simulink model "cruise_model_expanded"  (R2017a)
settings: Solver=VariableStepAuto  StartTime=0.0  StopTime=700  RelTol=1e-3
model workspace: external: MAT-File cruise_model_expanded_params.mat (data not in the file)
undefined symbols (not defined in the file or in its folder): D, DOutMax, DOutMin, I, InitialConditionForFilter, InitialConditionForIntegrator, IOutMax, IOutMin, N, NOutMax, NOutMin, P, POutMax, POutMin, SampleTime, SumDOutMax, SumDOutMin, SumOutMax, SumOutMin
libraries: simulink x1
settings Model: Creator=root  LastModifiedBy=nikhil

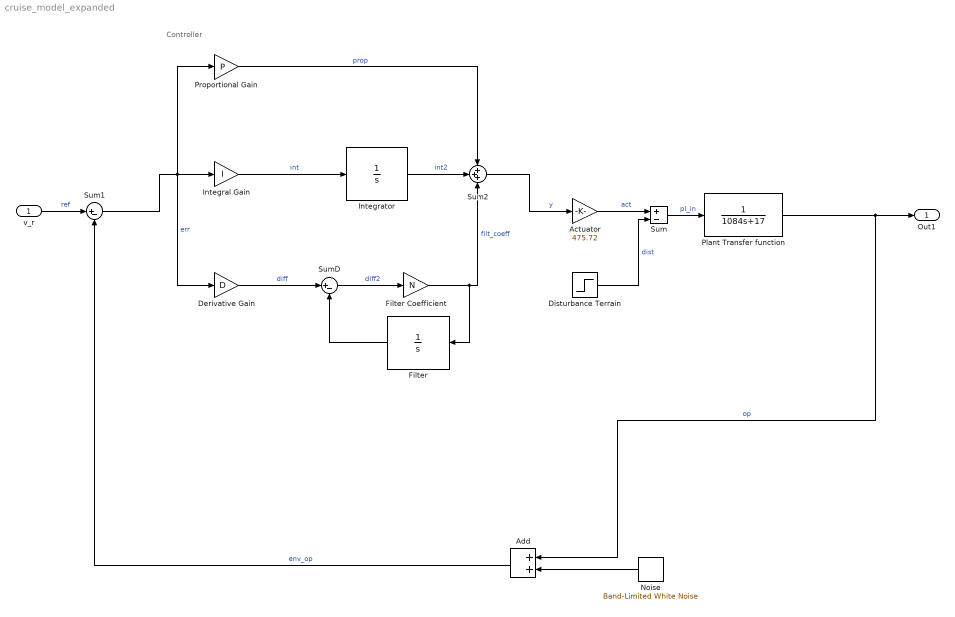
== system cruise_model_expanded ==
  note: Controller
  v_r : Inport
  " Noise" : simulink/Sources/Band-Limited White Noise  Cov=[0.01]  Ts=0.1  seed=[23341]
  Actuator : Gain  Gain=475.72
  Add : Sum
  Derivative Gain : Gain  DisableCoverage=on  Gain=D  ParamMin=DParamMin  ParamMax=DParamMax  OutMin=DOutMin  OutMax=DOutMax  SampleTime=SampleTime
  Disturbance Terrain : Step  Time=350  After=475.72*9.81*sin(pi/45)  SampleTime=0
  Filter : Integrator  DisableCoverage=on  InitialCondition=InitialConditionForFilter
  Filter Coefficient : Gain  Gain=N  ParamMin=NParamMin  ParamMax=NParamMax  OutMin=NOutMin  OutMax=NOutMax  SampleTime=SampleTime
  Integral Gain : Gain  DisableCoverage=on  Gain=I  ParamMin=IParamMin  ParamMax=IParamMax  OutMin=IOutMin  OutMax=IOutMax  SampleTime=SampleTime
  Integrator : Integrator  InitialCondition=InitialConditionForIntegrator
  Plant Transfer function : TransferFcn  Denominator=[1084 17]
  Proportional Gain : Gain  Gain=P  ParamMin=PParamMin  ParamMax=PParamMax  OutMin=POutMin  OutMax=POutMax  SampleTime=SampleTime
  Sum : Sum  Inputs=+-
  Sum1 : Sum  Inputs=|+-
  Sum2 : Sum  Inputs=+++  OutMin=SumOutMin  OutMax=SumOutMax  SampleTime=SampleTime
  SumD : Sum  DisableCoverage=on  Inputs=|+-  OutMin=SumDOutMin  OutMax=SumDOutMax  SampleTime=SampleTime
  Out1 : Outport
  wires:
  Actuator/1 -> Sum/1  "act"
  Plant Transfer function/1 -> Out1/1, Add/1  "op"
  Disturbance Terrain/1 -> Sum/2  "dist"
  Sum/1 -> Plant Transfer function/1  "pl_in"
  " Noise"/1 -> Add/2
  Add/1 -> Sum1/2  "env_op"
  Sum1/1 -> Proportional Gain/1, Derivative Gain/1, Integral Gain/1  "err"
  v_r/1 -> Sum1/1  "ref"
  Derivative Gain/1 -> SumD/1  "diff"
  Filter/1 -> SumD/2
  Filter Coefficient/1 -> Sum2/3, Filter/1  "filt_coeff"
  Integral Gain/1 -> Integrator/1  "int"
  SumD/1 -> Filter Coefficient/1  "diff2"
  Proportional Gain/1 -> Sum2/1  "prop"
  Integrator/1 -> Sum2/2  "int2"
  Sum2/1 -> Actuator/1  "y"
